simulink model "differential"  (R2020a)
settings: Solver=VariableStepAuto  StartTime=0.0  StopTime=10.0  RelTol=1e-3
settings Model: Creator=11973  LastModifiedBy=11973

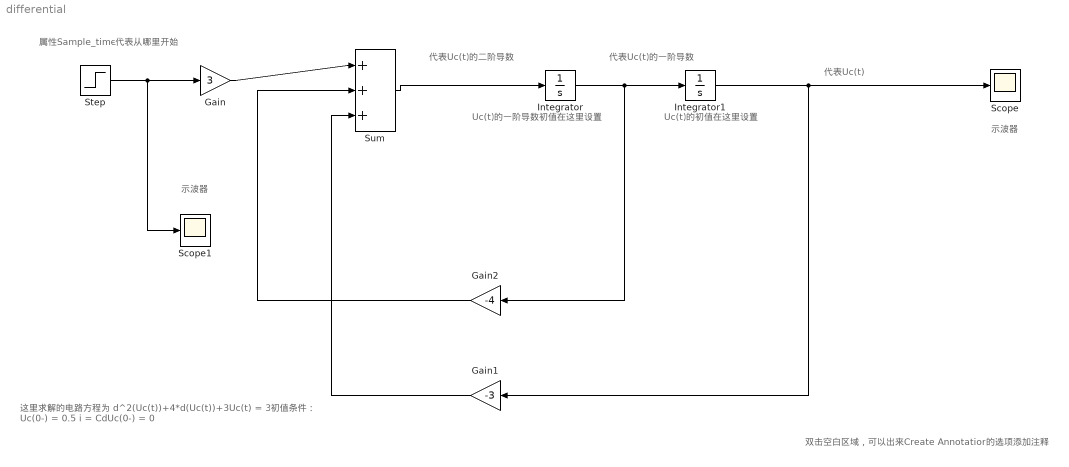
== system differential ==
  note: 示波器
  note: 代表Uc(t)
  note: 代表Uc(t)的一阶导数
  note: 代表Uc(t)的二阶导数
  note: Uc(t)的初值在这里设置
  note: Uc(t)的一阶导数初值在这里设置
  note: 这里求解的电路方程为
      | d^2(Uc(t))+4*d(Uc(t))+3Uc(t) = 3
      | 初值条件：
      | Uc(0-) = 0.5
      | i = CdUc(0-) = 0
  note: 属性Sample_time代表从哪里开始
  note: 双击空白区域，可以出来Create Annotation的选项添加注释
  note: 示波器
  Gain : Gain  Gain=3
  Gain1 : Gain  Gain=-3
  Gain2 : Gain  Gain=-4
  Integrator : Integrator
  Integrator1 : Integrator
  Scope : Scope
  Scope1 : Scope
  Step : Step  Time=0  SampleTime=0
  Sum : Sum  Inputs=|+++
  wires:
  Integrator/1 -> Gain2/1, Integrator1/1
  Integrator1/1 -> Scope/1, Gain1/1
  Sum/1 -> Integrator/1
  Gain2/1 -> Sum/2
  Gain1/1 -> Sum/3
  Gain/1 -> Sum/1
  Step/1 -> Scope1/1, Gain/1
